simulink model "btdonghocbai1"  (R2022b)
settings: Solver=VariableStepAuto  StartTime=0.0  StopTime=10.0  RelTol=1e-3
settings Model: Creator=admin  LastModifiedBy=admin

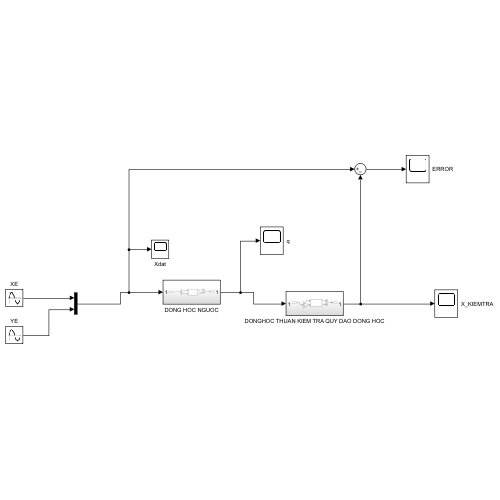
[thumbnail: Simulink's stored preview of the top-level diagram]
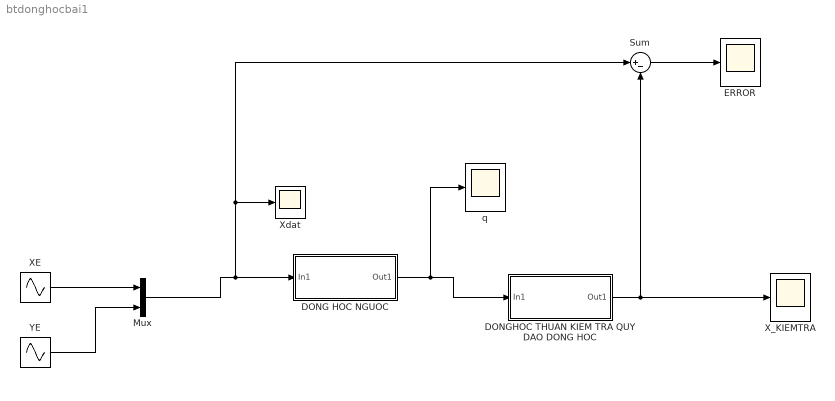
== system btdonghocbai1 ==
  DONG HOC NGUOC : Subsystem
  DONGHOC THUAN KIEM TRA QUY DAO DONG HOC : Subsystem
  ERROR : Scope
  Mux : Mux  Inputs=2
  Sum : Sum  Inputs=|+-
  XE : Sin  Amplitude=1.231  SampleTime=0
  X_KIEMTRA : Scope
  Xdat : Scope
  YE : Sin  Amplitude=1.43  SampleTime=0
  q : Scope
  wires:
  XE/1 -> Mux/1
  YE/1 -> Mux/2
  Mux/1 -> Sum/1, Xdat/1, DONG HOC NGUOC/1(In1)
  DONG HOC NGUOC/1(Out1) -> q/1, DONGHOC THUAN KIEM TRA QUY DAO DONG HOC/1(In1)
  DONGHOC THUAN KIEM TRA QUY DAO DONG HOC/1(Out1) -> X_KIEMTRA/1, Sum/2
  Sum/1 -> ERROR/1

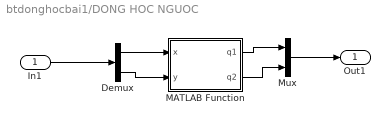
== system btdonghocbai1/DONG HOC NGUOC ==
  In1 : Inport
  Demux : Demux  Outputs=2
  MATLAB Function : MATLAB Function  TreatAsAtomicUnit=on
  Mux : Mux  Inputs=2
  Out1 : Outport
  wires:
  Demux/1 -> MATLAB Function/1(x)
  Demux/2 -> MATLAB Function/2(y)
  In1/1 -> Demux/1
  MATLAB Function/1(q1) -> Mux/1
  MATLAB Function/2(q2) -> Mux/2
  Mux/1 -> Out1/1

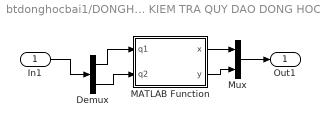
== system btdonghocbai1/DONGHOC THUAN KIEM TRA QUY DAO DONG HOC ==
  In1 : Inport
  Demux : Demux  Outputs=2
  MATLAB Function : MATLAB Function  TreatAsAtomicUnit=on
  Mux : Mux  Inputs=2
  Out1 : Outport
  wires:
  In1/1 -> Demux/1
  Demux/1 -> MATLAB Function/1(q1)
  Demux/2 -> MATLAB Function/2(q2)
  MATLAB Function/1(x) -> Mux/1
  MATLAB Function/2(y) -> Mux/2
  Mux/1 -> Out1/1

== matlab function btdonghocbai1/DONGHOC THUAN KIEM TRA QUY DAO DONG HOC/MATLAB Function ==
  data: x output; q1 input; y output; q2 input
function [x,y]=fcn(q1,q2)
L1=1;
L2=1;
x=L1*cos(q1)+L2*cos(q1+q2);
y=L1*sin(q1)+L2*sin(q1+q2);

end

== matlab function btdonghocbai1/DONG HOC NGUOC/MATLAB Function ==
  data: x input; q1 output; y input; q2 output

function [q1,q2]=fcn(x,y)
L1=1;
L2=1;
c2=(x^2+y^2-L1^2-L2^2)/(2*L1*L2);
q2=(-acos(c2));
D=x^2+y^2;
Dx=(L1+L2*cos(q2))*x+L2*sin(q2)*y;
c1=Dx/D;
q1=acos(c1);
end
